simulink model "exp35"  (R2022a)
settings: Solver=FixedStepAuto  StartTime=0.0  StopTime=sim_T  FixedStep=1e-10  RelTol=1e-3
undefined symbols (not defined in the file): AT, BT, CT, DT
settings Model: Creator=leon  LastModifiedBy=leon

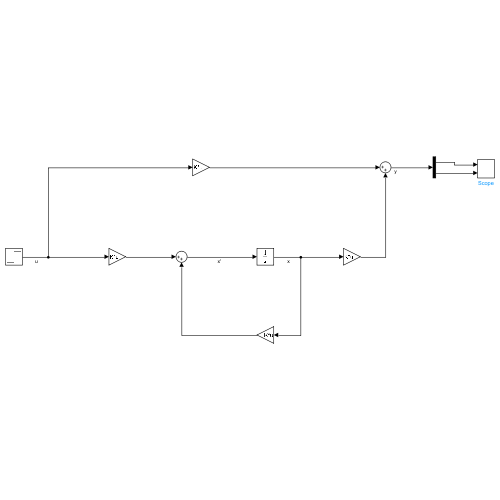
[thumbnail: Simulink's stored preview of the top-level diagram]
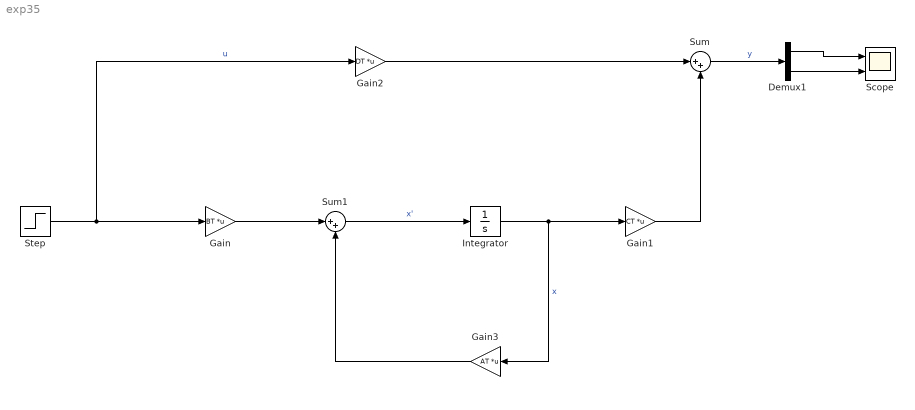
== system exp35 ==
  Demux1 : Demux  Outputs=2
  Gain : Gain  Gain=BT  Multiplication=Matrix(K*u)
  Gain1 : Gain  Gain=CT  Multiplication=Matrix(K*u)
  Gain2 : Gain  Gain=DT  Multiplication=Matrix(K*u)
  Gain3 : Gain  Gain=AT  Multiplication=Matrix(K*u)
  Integrator : Integrator
  Scope : Scope  NumInputPorts=2
  Step : Step  Time=0  SampleTime=0
  Sum : Sum  Inputs=|++
  Sum1 : Sum  Inputs=|++
  wires:
  Step/1 -> Gain2/1, Gain/1  "u"
  Integrator/1 -> Gain3/1, Gain1/1  "x"
  Gain3/1 -> Sum1/2
  Gain/1 -> Sum1/1
  Sum1/1 -> Integrator/1  "x'"
  Gain2/1 -> Sum/1
  Gain1/1 -> Sum/2
  Sum/1 -> Demux1/1  "y"
  Demux1/1 -> Scope/1
  Demux1/2 -> Scope/2
